simulink model "asimgenj3sat"  (R2015a)
settings: Solver=ode45  StartTime=0.0  StopTime=10.0  RelTol=1e-3
values from neighbouring files (symbols this model uses):
  Kimiz4 = x(2)    [geneticj3sat.m]
  Kpmiz4 = x(1)    [geneticj3sat.m]
settings Model: Creator=PC  LastModifiedBy=PC

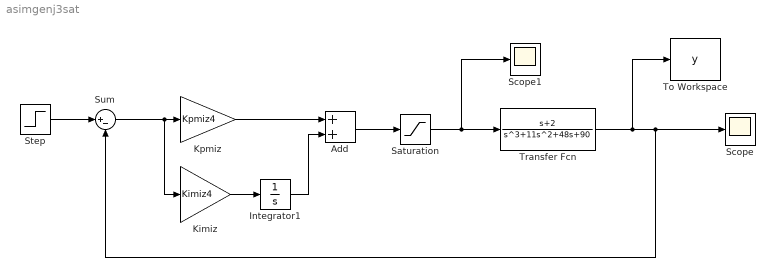
== system asimgenj3sat ==
  Add : Sum
  Integrator1 : Integrator
  Kimiz : Gain  Gain=Kimiz4
  Kpmiz : Gain  Gain=Kpmiz4
  Saturation : Saturate  UpperLimit=90  LowerLimit=0
  Scope : Scope
      settings: TimeRange=10  DataFormat=Structure  MaxDataPoints=20000  Decimation=5
  Scope1 : Scope
  Step : Step  SampleTime=0
  Sum : Sum  Inputs=|+-
  To Workspace : ToWorkspace  VariableName=y  SampleTime=-1
  Transfer Fcn : TransferFcn  Numerator=[1 2]  Denominator=[1 11 48 90]
  wires:
  Sum/1 -> Kpmiz/1, Kimiz/1
  Step/1 -> Sum/1
  Kimiz/1 -> Integrator1/1
  Integrator1/1 -> Add/2
  Kpmiz/1 -> Add/1
  Transfer Fcn/1 -> To Workspace/1, Sum/2, Scope/1
  Add/1 -> Saturation/1
  Saturation/1 -> Scope1/1, Transfer Fcn/1
